simulink model "TCMSSystem"  (R2019b)
settings: configuration reference "ConfigSet_TCMSSystem_Reference" (kept outside this file)
model workspace (MAT data in the model file):
  Prm_TCMSSystem : Simulink.Parameter (value not decoded)
  SampleTime = 0.05
symbols that are objects in the model workspace (value not decoded): Prm_TCMSSystem
undefined symbols (not defined in the file): ADDIntervention, AK1Status, AK2Status, AKContactorStatus, AllDoorsClosed, AllLeftDoorsClosed, AllRightDoorsClosed, APS1Fault, APS1Isolated, APS1OutputVoltage, APS1Status, APS2Fault, APS2Isolated, APS2OutputVoltage, APS2Status, APSKAKContactor, ASCOEnd1, ASCOEnd2, ATBMode, ATCBypassMode, ATCStatusNotOK, ATOMode, ATPLowSpeedCutoutStatus, ATPMode, AuxCompressor, BatteryCurrent, BatteryIsolationContactor, BatteryTemperature, BatteryVoltage, BCG1Fault, BCG1Isolated, BCG1IsolationFailed, BCG1OutputCurrent, BCG1Status, BCG2Fault, BCG2Isolated, BCG2OutputCurrent, BCG2Status, BCGOutputVoltage, BECU1AxleLockedWheelSet1, BECU2AxleLockedWheelSet2, BECUFaulty, BECUMajorFault, BECUMinorFault, BECUStatus, BIC1Inside, BIC1Outside, BIC2Inside, BIC2Outside, Bogie, Bogie1WSPStatus, Bogie2WSPStatus, BogieFaulty, BogieIsolationStatus, BogieSupportedMass, BrakeCylinderPressureGauge, BrakeLoopCBTripped, BrakeLoopOpenTL, BrakeTrainLineStatus, BrakingDemand ... (+215)
libraries: TimersLib x257, simulink x137, LatchesLib x42, VectorOperationsLib x15, TestBenchLib x12, MathOperationsLib x2, FiltersLib x1
(part 4 of 16)

== system TCMSSystem/TCMSSystemPerVehicle/EnabledTCMSVehicle/TCMSPneumatics/PneumaticControl ==
  In Bus Element1 : Inport  PortName=WireStates  Element=TractionBrakingTrainWire.BrakingCommand
  In Bus Element : Inport  Port=2  PortName=IOControl  Element=ASCOEnd1
  In Bus Element2 : Inport  Port=2  PortName=IOControl  Element=ASCOEnd2
  In Bus Element3 : Inport  Port=2  PortName=IOControl  Element=HornManuallyIsolated
  In Bus Element4 : Inport  Port=2  PortName=IOControl  Element=BIC1Inside
  In Bus Element5 : Inport  Port=2  PortName=IOControl  Element=BIC1Outside
  In Bus Element6 : Inport  Port=2  PortName=IOControl  Element=BIC2Inside
  In Bus Element7 : Inport  Port=2  PortName=IOControl  Element=BIC2Outside
  Bus Assignment : BusAssignment  AssignedSignals=BrakingDemand,ASCOEnd1,ASCOEnd2,HornManuallyIsolated,BIC1Inside,BIC1Outside,BIC2Inside,BIC2Outside
  Constant7 : Constant  Value=0  OutDataTypeStr=Bus: BD_TCMSSystem_Out_Vehicle_Control_PneumaticSystem
  Data Type Conversion{,1..6} (7 alike) : DataTypeConversion
  NOT{,1..6} (7 alike) : Logic  Operator=NOT  AllPortsSameDT=off  OutDataTypeStr=boolean
  Control : Outport
  wires:
  Constant7/1 -> Bus Assignment/1  "Control"
  Bus Assignment/1 -> Control/1  "Control"
  In Bus Element1/1 -> Bus Assignment/2
  In Bus Element2/1 -> NOT1/1
  In Bus Element/1 -> NOT/1
  NOT/1 -> Data Type Conversion1/1
  NOT1/1 -> Data Type Conversion/1
  Data Type Conversion/1 -> Bus Assignment/4
  Data Type Conversion1/1 -> Bus Assignment/3
  In Bus Element3/1 -> NOT2/1
  Data Type Conversion2/1 -> Bus Assignment/5
  NOT2/1 -> Data Type Conversion2/1
  NOT3/1 -> Data Type Conversion3/1
  Data Type Conversion3/1 -> Bus Assignment/6
  Data Type Conversion4/1 -> Bus Assignment/7
  NOT4/1 -> Data Type Conversion4/1
  NOT5/1 -> Data Type Conversion5/1
  Data Type Conversion5/1 -> Bus Assignment/8
  Data Type Conversion6/1 -> Bus Assignment/9
  NOT6/1 -> Data Type Conversion6/1
  In Bus Element4/1 -> NOT3/1
  In Bus Element5/1 -> NOT4/1
  In Bus Element6/1 -> NOT5/1
  In Bus Element7/1 -> NOT6/1

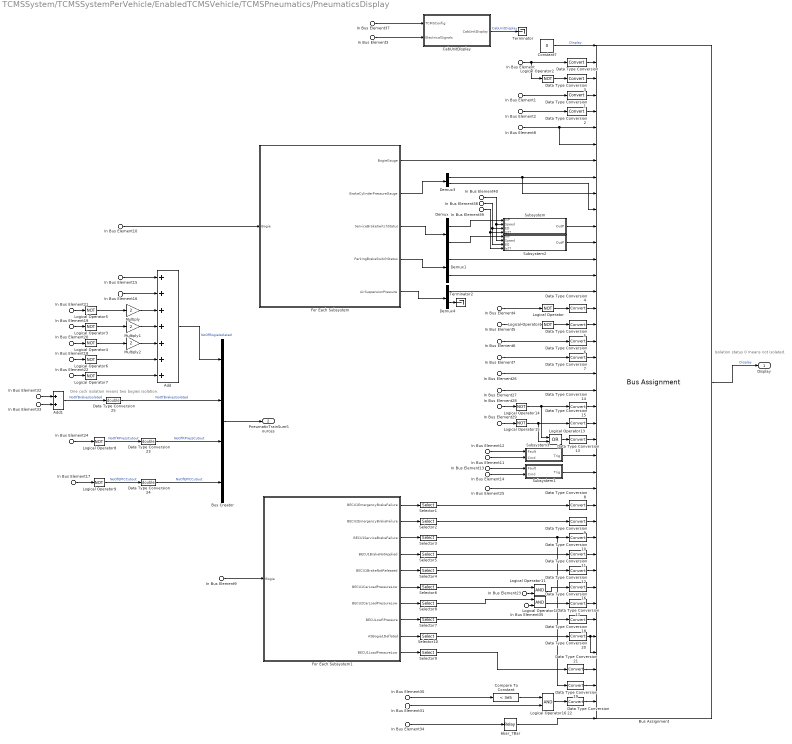
== system TCMSSystem/TCMSSystemPerVehicle/EnabledTCMSVehicle/TCMSPneumatics/PneumaticsDisplay ==
  note: One cock isolation means two bogies isolation.
  note: Isolation status 0 means not isolated.
  In Bus Element37 : Inport  PortName=TCMSSystemVehicleConfig
  In Bus Element39 : Inport  PortName=TCMSSystemVehicleConfig  Element=IsTCar
  In Bus Element3 : Inport  Port=2  PortName=ElectricalSignals
  In Bus Element : Inport  Port=2  PortName=ElectricalSignals  Element=ServiceBrakesReleased
  In Bus Element1 : Inport  Port=2  PortName=ElectricalSignals  Element=ParkBrakesReleased
  In Bus Element2 : Inport  Port=2  PortName=ElectricalSignals  Element=ParkBrakeApplication
  In Bus Element11 : Inport  Port=2  PortName=ElectricalSignals  Element=ParkBrakeApplyCommand
  In Bus Element14 : Inport  Port=2  PortName=ElectricalSignals  Element=ParkBrakeReleaseCommand
  In Bus Element8 : Inport  Port=3  PortName=PneumaticsSystem  Element=MainReservoirPressureGauge
  In Bus Element34 : Inport  Port=3  PortName=PneumaticsSystem  Element=MainReservoirPressureGauge
  In Bus Element10 : Inport  Port=3  PortName=PneumaticsSystem  Element=Bogie
  In Bus Element9 : Inport  Port=3  PortName=PneumaticsSystem  Element=Bogie
  In Bus Element25 : Inport  Port=3  PortName=PneumaticsSystem  Element=BrakeDemandSignalFailure
  In Bus Element30 : Inport  Port=3  PortName=PneumaticsSystem  Element=PantographPressure
  In Bus Element4 : Inport  Port=4  PortName=IOControl  Element=ASCOEnd1
  In Bus Element18 : Inport  Port=4  PortName=IOControl  Element=ASCOEnd1
  In Bus Element5 : Inport  Port=4  PortName=IOControl  Element=ASCOEnd2
  In Bus Element22 : Inport  Port=4  PortName=IOControl  Element=ASCOEnd2
  In Bus Element{6,15,26,32} (4 alike) : Inport  Port=4  PortName=IOControl  Element=Bogie1IsolationCmd
  In Bus Element{7,16,27,33} (4 alike) : Inport  Port=4  PortName=IOControl  Element=Bogie2IsolationCmd
  In Bus Element19 : Inport  Port=4  PortName=IOControl  Element=EPIC
  In Bus Element17 : Inport  Port=4  PortName=IOControl  Element=EPIC
  In Bus Element20 : Inport  Port=4  PortName=IOControl  Element=SR
  In Bus Element24 : Inport  Port=4  PortName=IOControl  Element=SR
  In Bus Element21 : Inport  Port=4  PortName=IOControl  Element=ASIsolationCock
  In Bus Element28 : Inport  Port=4  PortName=IOControl  Element=ParkBrakeIsolationCockBogie1
  In Bus Element29 : Inport  Port=4  PortName=IOControl  Element=ParkBrakeIsolationCockBogie2
  In Bus Element12 : Inport  Port=5  PortName=PneumaticFaults  Element=ParkingBrakeApplicationFailure
  In Bus Element13 : Inport  Port=5  PortName=PneumaticFaults  Element=ParkingBrakeReleaseFailure
  In Bus Element31 : Inport  Port=5  PortName=PneumaticFaults  Element=PantographPipeLowPressure
  In Bus Element23 : Inport  Port=5  PortName=PneumaticFaults  Element=BECU1CarLoadPressureLow
  In Bus Element35 : Inport  Port=5  PortName=PneumaticFaults  Element=BECU2CarLoadPressureLow
  In Bus Element38 : Inport  Port=6  PortName=TractionBrakingFB  Element=EDBrakingCommand
  In Bus Element40 : Inport  Port=7  PortName=Dynamics  Element=VehicleSpeed
  6bar_7Bar : Relay  OnSwitchValue=700000  OffSwitchValue=600000  OnOutputValue=0  OffOutputValue=1
  Add : Sum  Inputs=+++++++
  Add1 : Sum
  Bus Assignment : BusAssignment  AssignedSignals=AllServiceBrakesReleased,ServiceBrakesApplied,AllParkBrakesReleased,ParkBrakeApplied,MainReservoirPressureGauge,MainPipePressure,Bogie,BrakeCylinderPressure,Bogie1BrakeCylinderPressure,Bogie2BrakeCylinderPressure,Bogie1ServiceBrakeStatus,Bogie2ServiceBrakeStatus,Bogie1ParkingBrakeStatus,Bogie2ParkingBrakeStatus,AirSuspensionPressure,Bogie1SUSPStatus,Bogie2SUSPStatus,Bogie1IsolationStatus,Bogie2IsolationStatus,Bogie1ServiceBrakeIsolated,Bogie2ServiceBrakeIsolated,Bogie1ParkingBrakeIsolated,Bogie2ParkingBrakeIsolated,ParkBrakeIsolated,ParkBrakeApplyFailure,ParkBrakeReleaseFailure,BrakeDemandSignalFailure,BECU1EmergencyBrakeFailure,BECU2EmergencyBrakeFailure,BECU1ServiceBrakeFailure,BECU1BrakeNotApplied,BECU1BrakeNotReleased,BECU1CarLoadPressureLow,BECU2CarLoadPressureLow,BECULowRPressure,AirSuspensionBogie1Deflated,Bogie1SUSPFault,BECU1LoadPressureLow,Bogie1ServiceBrakeFault,PantographPipePressureLow,MainReservoirPressureLow
  Bus Creator : BusCreator  Inputs=4  OutDataTypeStr=Bus: BD_TCMSSystem_Wires_PneumaticTrainSum  NonVirtualBus=on
  CabUnitDisplay : Subsystem
  Compare To Constant : simulink/Logic and Bit Operations/Compare To Constant  relop=<  const=3e5  OutDataTypeStr=boolean
  Constant7 : Constant  Value=0  OutDataTypeStr=Bus: BD_TCMSSystem_Out_Vehicle_Display_PneumaticsSystem
  Data Type Conversion{,1..22} (23 alike) : DataTypeConversion
  Data Type Conversion23 : DataTypeConversion  OutDataTypeStr=double
  Data Type Conversion24 : DataTypeConversion  OutDataTypeStr=double
  Data Type Conversion25 : DataTypeConversion  OutDataTypeStr=double
  Demux{,1,3..4} (4 alike) : Demux  Outputs=2
  For Each Subsystem : Subsystem  TreatAsAtomicUnit=on
  For Each Subsystem1 : Subsystem  TreatAsAtomicUnit=on
  Logical Operator{,1..9,14..15} (12 alike) : Logic  Operator=NOT  AllPortsSameDT=off  OutDataTypeStr=boolean
  Logical Operator10 : Logic  AllPortsSameDT=off  OutDataTypeStr=boolean
  Logical Operator11 : Logic  AllPortsSameDT=off  OutDataTypeStr=boolean
  Logical Operator13 : Logic  Operator=OR  AllPortsSameDT=off  OutDataTypeStr=boolean
  Logical Operator16 : Logic  AllPortsSameDT=off  OutDataTypeStr=boolean
  Multiply : Gain  Gain=2
  Multiply1 : Gain  Gain=2
  Multiply2 : Gain  Gain=2
  Selector{1..10} (10 alike) : Selector  InputPortWidth=2  IndexOptions=Index vector (dialog)  Indices=[1]  OutputSizes=1
  Subsystem : Subsystem
  Subsystem1 : Subsystem
  Subsystem2 : Subsystem
  Subsystem3 : Subsystem
  Terminator : Terminator
  Terminator2 : Terminator
  Display : Outport
  PneumaticTrainSumSources : Outport  Port=2
  wires:
  In Bus Element/1 -> Logical Operator2/1, Data Type Conversion/1
  In Bus Element1/1 -> Data Type Conversion1/1
  CabUnitDisplay/1(CabUnitDisplay) -> Terminator/1  "CabUnitDisplay"
  In Bus Element3/1 -> CabUnitDisplay/2(ElectricalSignals)
  In Bus Element37/1 -> CabUnitDisplay/1(TCMSConfig)
  Bus Assignment/1 -> Display/1  "Display"
  Constant7/1 -> Bus Assignment/1  "Display"
  In Bus Element2/1 -> Data Type Conversion2/1
  In Bus Element10/1 -> For Each Subsystem/1(Bogie)
  Logical Operator2/1 -> Data Type Conversion3/1
  Data Type Conversion/1 -> Bus Assignment/2
  Data Type Conversion1/1 -> Bus Assignment/4
  Data Type Conversion2/1 -> Bus Assignment/5
  Data Type Conversion3/1 -> Bus Assignment/3
  For Each Subsystem/3(ServiceBrakeSwitchStatus) -> Demux/1
  For Each Subsystem/4(ParkingBrakeSwitchStatus) -> Demux1/1
  In Bus Element8/1 -> Bus Assignment/7, Bus Assignment/6
  For Each Subsystem/5(AirSuspensionPressure) -> Demux4/1
  Demux4/2 -> Terminator2/1
  Demux/2 -> Subsystem2/1(InP)
  Demux1/1 -> Bus Assignment/14
  Demux1/2 -> Bus Assignment/15
  In Bus Element4/1 -> Logical Operator/1
  In Bus Element5/1 -> Logical Operator1/1
  Demux3/2 -> Bus Assignment/11
  Demux4/1 -> Bus Assignment/16
  Demux3/1 -> Bus Assignment/10, Bus Assignment/9
  Logical Operator/1 -> Data Type Conversion4/1
  Logical Operator1/1 -> Data Type Conversion5/1
  Bus Creator/1 -> PneumaticTrainSumSources/1
  Add/1 -> Bus Creator/1  "NoOfBogieIsolated"
  Data Type Conversion4/1 -> Bus Assignment/17
  Data Type Conversion5/1 -> Bus Assignment/18
  For Each Subsystem/1(BogieGauge) -> Bus Assignment/8
  For Each Subsystem/2(BrakeCylinderPressureGauge) -> Demux3/1
  Subsystem3/1(Trig) -> Bus Assignment/26
  Subsystem1/1(Trig) -> Bus Assignment/27
  In Bus Element13/1 -> Subsystem1/1(Fault)
  In Bus Element12/1 -> Subsystem3/1(Fault)
  In Bus Element14/1 -> Subsystem1/2(Cmd)
  In Bus Element11/1 -> Subsystem3/2(Cmd)
  In Bus Element15/1 -> Add/1
  In Bus Element16/1 -> Add/2
  Logical Operator5/1 -> Multiply/1
  In Bus Element21/1 -> Logical Operator5/1
  Logical Operator3/1 -> Multiply1/1
  Logical Operator4/1 -> Multiply2/1
  In Bus Element20/1 -> Logical Operator4/1
  In Bus Element19/1 -> Logical Operator3/1
  Multiply/1 -> Add/3
  Multiply1/1 -> Add/4
  Multiply2/1 -> Add/5
  Data Type Conversion6/1 -> Bus Assignment/19
  In Bus Element6/1 -> Data Type Conversion6/1
  In Bus Element7/1 -> Data Type Conversion7/1
  Data Type Conversion7/1 -> Bus Assignment/20
  In Bus Element18/1 -> Logical Operator6/1
  In Bus Element22/1 -> Logical Operator7/1
  In Bus Element25/1 -> Bus Assignment/28
  In Bus Element9/1 -> For Each Subsystem1/1(Bogie)
  For Each Subsystem1/1(BECU1EmergencyBrakeFailure) -> Selector1/1
  For Each Subsystem1/2(BECU2EmergencyBrakeFailure) -> Selector2/1
  For Each Subsystem1/3(BECU1ServiceBrakeFailure) -> Selector3/1
  For Each Subsystem1/4(BECU1BrakeNotApplied) -> Selector5/1
  For Each Subsystem1/5(BECU1BrakeNotReleased) -> Selector4/1
  Selector1/1 -> Data Type Conversion8/1
  Selector2/1 -> Data Type Conversion9/1
  Selector3/1 -> Data Type Conversion10/1, Data Type Conversion19/1
  Selector5/1 -> Data Type Conversion11/1
  Selector4/1 -> Data Type Conversion12/1
  Data Type Conversion8/1 -> Bus Assignment/29
  Data Type Conversion9/1 -> Bus Assignment/30
  Data Type Conversion10/1 -> Bus Assignment/31
  Data Type Conversion11/1 -> Bus Assignment/32
  Data Type Conversion12/1 -> Bus Assignment/33
  In Bus Element27/1 -> Bus Assignment/22
  In Bus Element28/1 -> Logical Operator14/1
  In Bus Element29/1 -> Logical Operator15/1
  Logical Operator13/1 -> Data Type Conversion13/1
  Data Type Conversion13/1 -> Bus Assignment/25
  Logical Operator14/1 -> Data Type Conversion14/1, Logical Operator13/1
  Logical Operator15/1 -> Logical Operator13/2, Data Type Conversion15/1
  Data Type Conversion14/1 -> Bus Assignment/23
  Data Type Conversion15/1 -> Bus Assignment/24
  Data Type Conversion17/1 -> Bus Assignment/35
  For Each Subsystem1/8(BECULowRPressure) -> Selector7/1
  For Each Subsystem1/7(BECU2CarLoadPressureLow) -> Selector8/1
  For Each Subsystem1/6(BECU1CarLoadPressureLow) -> Selector6/1
  Selector7/1 -> Data Type Conversion18/1
  Logical Operator10/1 -> Data Type Conversion17/1
  Selector6/1 -> Logical Operator11/1
  Data Type Conversion16/1 -> Bus Assignment/34
  Data Type Conversion18/1 -> Bus Assignment/36
  Data Type Conversion19/1 -> Bus Assignment/40
  Data Type Conversion21/1 -> Bus Assignment/39
  Selector10/1 -> Data Type Conversion20/1
  Selector9/1 -> Data Type Conversion21/1
  For Each Subsystem1/9(ASBogie1Deflated) -> Selector10/1
  For Each Subsystem1/10(BECU1LoadPressureLow) -> Selector9/1
  Data Type Conversion20/1 -> Bus Assignment/38, Bus Assignment/37
  Logical Operator16/1 -> Data Type Conversion22/1
  In Bus Element30/1 -> Compare To Constant/1
  Compare To Constant/1 -> Logical Operator16/1
  In Bus Element31/1 -> Logical Operator16/2
  Data Type Conversion22/1 -> Bus Assignment/41
  Logical Operator6/1 -> Add/6
  Logical Operator7/1 -> Add/7
  In Bus Element34/1 -> 6bar_7Bar/1
  6bar_7Bar/1 -> Bus Assignment/42
  In Bus Element24/1 -> Logical Operator8/1
  Data Type Conversion23/1 -> Bus Creator/3  "NoOfRPressCutout"
  In Bus Element17/1 -> Logical Operator9/1
  Data Type Conversion24/1 -> Bus Creator/4  "NoOfEPICCutout"
  Logical Operator8/1 -> Data Type Conversion23/1  "NoOfRPressCutout"
  Logical Operator9/1 -> Data Type Conversion24/1  "NoOfEPICCutout"
  In Bus Element32/1 -> Add1/1
  In Bus Element33/1 -> Add1/2
  Add1/1 -> Data Type Conversion25/1  "NoOfBrakesIsolated"
  Data Type Conversion25/1 -> Bus Creator/2  "NoOfBrakesIsolated"
  Logical Operator11/1 -> Data Type Conversion16/1
  Selector8/1 -> Logical Operator10/1
  In Bus Element23/1 -> Logical Operator11/2
  In Bus Element35/1 -> Logical Operator10/2
  In Bus Element26/1 -> Bus Assignment/21
  Demux/1 -> Subsystem/1(InP)
  In Bus Element40/1 -> Subsystem2/2(Speed), Subsystem/2(Speed)
  In Bus Element38/1 -> Subsystem2/3(ED), Subsystem/3(ED)
  In Bus Element39/1 -> Subsystem/4(IsT?), Subsystem2/4(IsT?)
  Subsystem/1(OutP) -> Bus Assignment/12
  Subsystem2/1(OutP) -> Bus Assignment/13

== system TCMSSystem/TCMSSystemPerVehicle/EnabledTCMSVehicle/TCMSStatus/TCMSSystemDisplay ==
  TCMSSystemVehicleConfig : Inport
  In Bus Element2 : Inport  Port=2  PortName=DisplayControl  Element=HornIsolate
  In Bus Element1 : Inport  Port=3  PortName=TCMSFaults  Element=CCUCommunicationError
  In Bus Element3 : Inport  Port=3  PortName=TCMSFaults  Element=RIO1Fault
  In Bus Element4 : Inport  Port=3  PortName=TCMSFaults  Element=RIO1RIO2Fault
  In Bus Element5 : Inport  Port=3  PortName=TCMSFaults  Element=ERFault
  In Bus Element7 : Inport  Port=4  PortName=ElectricalIn  Element=MCDR
  AND1 : Logic  AllPortsSameDT=off  OutDataTypeStr=boolean
  Bus Assignment : BusAssignment  AssignedSignals=ConsistSwitchStatusA,ConsistSwitchStatusB,ConsistSwitchStatusC,TrainEthernetRepeaterStatus,TrainBackboneNodeStatus,ECNALGStatus,RemoteHornIsolated,CCUFault,RIO1Fault,RIO1Status,RIO2Status,ERFault,RIO1RIO2Fault
  Bus Selector1 : BusSelector  OutputSignals=HasCab
  Constant : Constant
  Constant1 : Constant
  Constant2 : Constant  Value=0
  Constant7 : Constant  Value=0  OutDataTypeStr=Bus: BD_TCMSSystem_Out_Vehicle_Display_TCMSSystem
  Data Type Conversion : DataTypeConversion
  Data Type Conversion2 : DataTypeConversion
  Switch : Switch  Criteria=u2 > Threshold
  Display : Outport
  wires:
  Constant7/1 -> Bus Assignment/1  "Display"
  Bus Assignment/1 -> Display/1  "Display"
  Constant/1 -> Bus Assignment/7, Bus Assignment/5, Bus Assignment/4, Bus Assignment/3, Bus Assignment/2
  TCMSSystemVehicleConfig/1 -> Bus Selector1/1
  Bus Selector1/1 -> AND1/1  "<HasCab>"
  In Bus Element7/1 -> Data Type Conversion/1
  Data Type Conversion/1 -> Bus Assignment/6
  In Bus Element2/1 -> Bus Assignment/8
  In Bus Element1/1 -> AND1/2
  In Bus Element3/1 -> Bus Assignment/10
  In Bus Element5/1 -> Bus Assignment/13
  AND1/1 -> Data Type Conversion2/1
  Data Type Conversion2/1 -> Bus Assignment/9
  In Bus Element4/1 -> Bus Assignment/14, Switch/2
  Switch/1 -> Bus Assignment/12, Bus Assignment/11
  Constant1/1 -> Switch/3
  Constant2/1 -> Switch/1

== system TCMSSystem/TCMSSystemPerVehicle/EnabledTCMSVehicle/TCMSTractionBraking/HoldingBrakeFB_ASDeflatedExtract ==
  In Bus Element1 : Inport  PortName=WireStates
  In Bus Element : Inport  PortName=WireStates  Element=HoldingBrakeStatus
  In Bus Element3 : Inport  Port=2  PortName=PneumaticsIn  Element=Bogie
  Bus Assignment : BusAssignment  AssignedSignals=HoldingBrakeStatus
  Compare To Constant : simulink/Logic and Bit Operations/Compare To Constant  relop=>=  const=0.8e5  OutDataTypeStr=boolean
  Data Type Conversion : DataTypeConversion
  Demux : Demux  Outputs=2
  For Each Subsystem : Subsystem  TreatAsAtomicUnit=on
  Logical Operator : Logic  AllPortsSameDT=off  OutDataTypeStr=boolean
  Selector : Selector  InputPortWidth=2  IndexOptions=Index vector (dialog)  Indices=1  OutputSizes=1
  Terminator : Terminator
  BusOut : Outport
  ASBogie1Deflated : Outport  Port=2
  wires:
  Bus Assignment/1 -> BusOut/1
  Logical Operator/1 -> Data Type Conversion/1
  In Bus Element1/1 -> Bus Assignment/1
  In Bus Element3/1 -> For Each Subsystem/1(Bogie)
  Demux/2 -> Terminator/1
  Demux/1 -> Compare To Constant/1
  Compare To Constant/1 -> Logical Operator/2
  In Bus Element/1 -> Logical Operator/1
  For Each Subsystem/1(BogieGauge) -> Demux/1
  Data Type Conversion/1 -> Bus Assignment/2
  Selector/1 -> ASBogie1Deflated/1
  For Each Subsystem/2(Out2) -> Selector/1

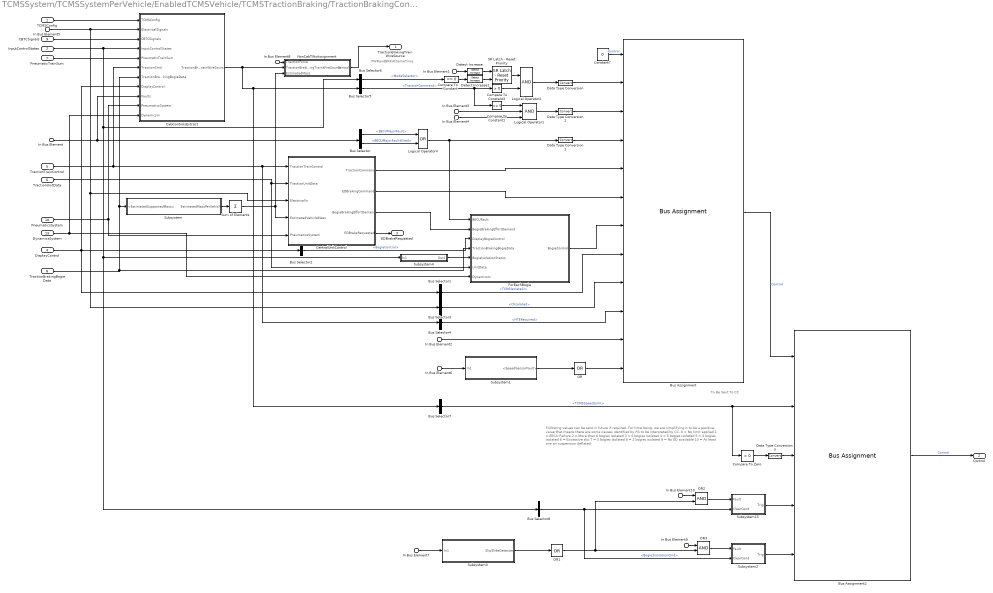
== system TCMSSystem/TCMSSystemPerVehicle/EnabledTCMSVehicle/TCMSTractionBraking/TractionBrakingControl ==
  note: To Be Sent To CC
  note: Following values can be sent in future if required. For time being, we are simplifying it to be a positive value
      | that means there are some causes identified by RS to be interpreted by CC.
      | 0 = No limit applied
      | 1 = EBCU Failure
      | 2 = More than 6 bogies isolated
      | 3 = 6 bogies isolated
      | 4 = 5 bogies isolated
      | 5 = 4 bogies isolated
      | 6 = Excessive slip
      | 7 = 3 bogies isolated
      | 8 = 2 bogies isolated
      | 9 = No ED available
      | 10 = At least one air suspension deflated
  note: PWRandBRKAtSameTime
  TCMSConfig : Inport
  InputControlStates : Inport  Port=2
  In Bus Element5 : Inport  Port=3  PortName=ElectricalSignals
  In Bus Element4 : Inport  Port=3  PortName=ElectricalSignals  Element=CabActive
  DisplayControl : Inport  Port=4
  TractionTrainControl : Inport  Port=5
  TractionUnitData : Inport  Port=6
  PneumaticTrainSum : Inport  Port=7
  TractionBrakingBogieData : Inport  Port=8
  CBTCSignals : Inport  Port=9
  PneumaticsSystem : Inport  Port=10
  In Bus Element : Inport  Port=11  PortName=Faults
  In Bus Element1 : Inport  Port=11  PortName=Faults  Element=BECUPWRAndBRKCmdAtSameTime
  In Bus Element3 : Inport  Port=11  PortName=Faults  Element=TractionCutModeSelectorInATPATOUTO
  In Bus Element2 : Inport  Port=12  PortName=TractionSystem  Element=VehicleDerailed
  In Bus Element6 : Inport  Port=12  PortName=TractionSystem  Element=Bogie
  In Bus Element7 : Inport  Port=12  PortName=TractionSystem  Element=Bogie
  In Bus Element8 : Inport  Port=12  PortName=TractionSystem  Element=TractionForce
  DynamicsSystem : Inport  Port=13
  In Bus Element9 : Inport  Port=14  PortName=VehicleFaults  Element=BECU2AxleLockedWheelSet2
  In Bus Element10 : Inport  Port=14  PortName=VehicleFaults  Element=BECU1AxleLockedWheelSet1
  Bus Assignment : BusAssignment  AssignedSignals=PWRandBRKBothApplied,TractionCutModeSelectorInATPATOUTO,BECUFaulty,TractionCommand,EDBrakingCommand,Bogie,TCMSIsolateCI,CIIsolated,HTERequired,VehicleDerailed,SpeedSensorFault
  Bus Assignment2 : BusAssignment  AssignedSignals=TCMSSpeedLimit,TCMSSpeedLimitCause,BECU1AxleLockedWheelSet1,BECU2AxleLockedWheelSet2
  Bus Selector : BusSelector  OutputSignals=BECUMajorFault,BECUMajorFaultWired
  Bus Selector1 : BusSelector  OutputSignals=TCMSIsolateCI
  Bus Selector2 : BusSelector  OutputSignals=BogieControl
  Bus Selector3 : BusSelector  OutputSignals=CIIsolated
  Bus Selector4 : BusSelector  OutputSignals=HTERequired
  Bus Selector5 : BusSelector  OutputSignals=TractionCommand
  Bus Selector6 : BusSelector  OutputSignals=ModeSelector
  Bus Selector7 : BusSelector  OutputSignals=TCMSSpeedLimit
  Bus Selector8 : BusSelector  OutputSignals=Bogie1IsolationCmd
  CabControlsExtract : Subsystem  TreatAsAtomicUnit=on
  CentralUnitControl : Subsystem  TreatAsAtomicUnit=on
  Compare To Constant : simulink/Logic and Bit Operations/Compare To Constant  relop===  const=0  OutDataTypeStr=boolean
  Compare To Constant1 : simulink/Logic and Bit Operations/Compare To Constant  relop===  const=0  OutDataTypeStr=boolean
  Compare To Constant3 : simulink/Logic and Bit Operations/Compare To Constant  relop=>  const=0  OutDataTypeStr=boolean
  Compare To Zero : simulink/Logic and Bit Operations/Compare To Zero  relop=>  OutDataTypeStr=boolean
  Constant7 : Constant  Value=0  OutDataTypeStr=Bus: BD_TCMSSystem_Out_Vehicle_Control_TractionBraking
  Data Type Conversion{,1..3} (4 alike) : DataTypeConversion
  Detect Increase : simulink/Logic and Bit Operations/Detect Increase  vinit=0.0  OutDataTypeStr=boolean
  Detect Increase1 : simulink/Logic and Bit Operations/Detect Increase  vinit=0.0  OutDataTypeStr=boolean
  ForEachBogie : Subsystem  TreatAsAtomicUnit=on
  Logical Operator1 : Logic  Inputs=3  AllPortsSameDT=off  OutDataTypeStr=boolean
  Logical Operator2 : Logic  AllPortsSameDT=off  OutDataTypeStr=boolean
  Logical Operator4 : Logic  Operator=OR  AllPortsSameDT=off  OutDataTypeStr=boolean
  NonCabTWsAssignment : Subsystem
  OR : Logic  Operator=OR  Inputs=1  AllPortsSameDT=off  OutDataTypeStr=boolean
  OR1 : Logic  Operator=OR  Inputs=1  AllPortsSameDT=off  OutDataTypeStr=boolean
  OR2 : Logic  AllPortsSameDT=off  OutDataTypeStr=boolean
  OR3 : Logic  AllPortsSameDT=off  OutDataTypeStr=boolean
  SR Latch - Reset Priority : LatchesLib/SR Latch - Reset Priority  initial_condition=0
      settings: SourceProductName=Latches
  Subsystem : Subsystem
  Subsystem1 : Subsystem
  Subsystem15 : Subsystem
  Subsystem2 : Subsystem
  Subsystem3 : Subsystem
  Subsystem4 : Subsystem
  Sum of Elements : Sum  Inputs=+
  TractionBrakingTrainWireSource : Outport
  Control : Outport  Port=2
  EDBrakeRequested : Outport  Port=3
  wires:
  Bus Assignment/1 -> Bus Assignment2/1  "Control"
  Constant7/1 -> Bus Assignment/1  "Control"
  TractionTrainControl/1 -> CabControlsExtract/6(TractionCmd), Bus Selector4/1, CentralUnitControl/1(TractionTrainControl)
  Bus Selector2/1 -> ForEachBogie/3(DisplayBogieControl)  "<BogieControl>"
  CentralUnitControl/3(BogieBrakingEffortDemand) -> ForEachBogie/2(BogieBrakingEffortDemand)
  TCMSConfig/1 -> CabControlsExtract/1(TCMSConfig)
  InputControlStates/1 -> Bus Selector8/1, Subsystem4/1(In1), Bus Selector6/1, CabControlsExtract/4(InputControlStates)
  In Bus Element5/1 -> Bus Selector3/1, CentralUnitControl/3(ElectricalIn), CabControlsExtract/2(ElectricalSignals)
  DisplayControl/1 -> Bus Selector1/1, CabControlsExtract/8(DisplayControl), Bus Selector2/1
  CBTCSignals/1 -> CabControlsExtract/3(CBTCSignals)
  CentralUnitControl/4(EDBrakeRequested) -> EDBrakeRequested/1
  CabControlsExtract/1(TractionBrakingTrainWireSource) -> NonCabTWsAssignment/2(TractionBrakingTrainWireSource), Bus Selector5/1, Bus Selector7/1
  TractionBrakingBogieData/1 -> CabControlsExtract/7(TractionBrakingBogieData), Subsystem/1(<EstimatedSupportedMass>), ForEachBogie/4(TractionBrakingBogieData)
  Subsystem/1(EstimatedMassPerVehicle) -> Sum of Elements/1
  Sum of Elements/1 -> CentralUnitControl/4(EstimatedVehicleMass), NonCabTWsAssignment/3(EstimatedMass)
  PneumaticTrainSum/1 -> CabControlsExtract/5(PneumaticTrainSum)
  In Bus Element/1 -> CabControlsExtract/9(Faults), Bus Selector/1
  PneumaticsSystem/1 -> CabControlsExtract/10(PneumaticsSystem), CentralUnitControl/5(PneumaticsSystem)
  Logical Operator4/1 -> Data Type Conversion1/1, ForEachBogie/1(BECUFault)
  Bus Selector/1 -> Logical Operator4/1  "<BECUMajorFault>"
  Bus Selector/2 -> Logical Operator4/2  "<BECUMajorFaultWired>"
  Data Type Conversion/1 -> Bus Assignment/2
  SR Latch - Reset Priority/1 -> Logical Operator2/1
  Detect Increase1/1 -> SR Latch - Reset Priority/2
  Logical Operator2/1 -> Data Type Conversion/1
  In Bus Element1/1 -> Detect Increase/1
  Compare To Constant3/1 -> Logical Operator2/2
  Detect Increase/1 -> SR Latch - Reset Priority/1
  Bus Selector6/1 -> Compare To Constant/1  "<ModeSelector>"
  Compare To Constant/1 -> Detect Increase1/1
  Bus Selector5/1 -> Compare To Constant1/1, Compare To Constant3/1  "<TractionCommand>"
  Compare To Constant1/1 -> Logical Operator1/1
  In Bus Element3/1 -> Logical Operator1/2
  ForEachBogie/1(BogieControl) -> Bus Assignment/7
  CentralUnitControl/2(EDBrakingCommand) -> Bus Assignment/6
  CentralUnitControl/1(TractionCommand) -> Bus Assignment/5
  Data Type Conversion1/1 -> Bus Assignment/4
  Logical Operator1/1 -> Data Type Conversion2/1
  In Bus Element2/1 -> Bus Assignment/11
  Bus Selector4/1 -> Bus Assignment/10  "<HTERequired>"
  Bus Selector3/1 -> Bus Assignment/9  "<CIIsolated>"
  Bus Selector1/1 -> Bus Assignment/8  "<TCMSIsolateCI>"
  Data Type Conversion2/1 -> Bus Assignment/3
  In Bus Element4/1 -> Logical Operator1/3
  Subsystem1/1(<SpeedSensorFault>) -> OR/1
  OR/1 -> Bus Assignment/12
  In Bus Element6/1 -> Subsystem1/1(In1)
  DynamicsSystem/1 -> CabControlsExtract/11(DynamicsIn), ForEachBogie/7(DynamicsIn)
  Bus Assignment2/1 -> Control/1  "Control"
  Compare To Zero/1 -> Data Type Conversion3/1
  Bus Selector7/1 -> Compare To Zero/1, Bus Assignment2/2  "<TCMSSpeedLimit>"
  In Bus Element8/1 -> NonCabTWsAssignment/1(TractionForce)
  NonCabTWsAssignment/1(Control) -> TractionBrakingTrainWireSource/1
  Data Type Conversion3/1 -> Bus Assignment2/3
  Subsystem15/1(Trig) -> Bus Assignment2/4
  Subsystem2/1(Trig) -> Bus Assignment2/5
  In Bus Element9/1 -> OR3/1
  In Bus Element10/1 -> OR2/1
  Bus Selector8/1 -> Subsystem15/2(ClearCond), Subsystem2/2(ClearCond)  "<Bogie1IsolationCmd>"
  In Bus Element7/1 -> Subsystem3/1(In1)
  OR1/1 -> OR2/2, OR3/2
  Subsystem3/1(SlipSlideDetected) -> OR1/1
  OR2/1 -> Subsystem15/1(Fault)
  OR3/1 -> Subsystem2/1(Fault)
  TractionUnitData/1 -> ForEachBogie/6(UnitData), CentralUnitControl/2(TractionUnitData)
  Subsystem4/1(Out1) -> ForEachBogie/5(BogieIsolationStatus)

== system TCMSSystem/TCMSSystemPerVehicle/EnabledTCMSVehicle/TCMSTractionBraking/TractionBrakingDataExtract ==
  note: Summing bogie outputs on each vehicle
  note: TCMSTractionVehicle
  TCMSSystemVehicleConfig : Inport
  In Bus Element : Inport  Port=2  PortName=TractionSystem  Element=Bogie
  In Bus Element2 : Inport  Port=2  PortName=TractionSystem  Element=TCU_KStatus
  In Bus Element3 : Inport  Port=2  PortName=TractionSystem  Element=TCU_AKStatus
  In Bus Element1 : Inport  Port=3  PortName=PneumaticsSystem  Element=Bogie
  AND : Logic  AllPortsSameDT=off  OutDataTypeStr=boolean
  AND1 : Logic  AllPortsSameDT=off  OutDataTypeStr=boolean
  Abs : Abs
  Abs1 : Abs
  Bus Creator : BusCreator  Inputs=13  OutDataTypeStr=Bus: BD_TCMSSystem_Wires_TBUnitSum  NonVirtualBus=on
  Bus Creator1 : BusCreator  Inputs=5  OutDataTypeStr=Bus: BD_TCMSSystem_Wires_TBUnitWire  NonVirtualBus=on
  Bus Selector : BusSelector  OutputSignals=NumberOfTractionBogies,NumberOfBrakingBogies
  Compare To Zero : simulink/Logic and Bit Operations/Compare To Zero  relop=>  OutDataTypeStr=boolean
  Compare To Zero1 : simulink/Logic and Bit Operations/Compare To Zero  relop=>  OutDataTypeStr=boolean
  Compare To Zero2 : simulink/Logic and Bit Operations/Compare To Zero  relop=>  OutDataTypeStr=boolean
  Data Type Conversion{,1..4} (5 alike) : DataTypeConversion
  Gain : Gain
  Gain1 : Gain
  NOT : Logic  Operator=NOT  AllPortsSameDT=off  OutDataTypeStr=boolean
  OR : Logic  Operator=OR  AllPortsSameDT=off  OutDataTypeStr=boolean
  OR1 : Logic  Operator=OR  Inputs=1  AllPortsSameDT=off  OutDataTypeStr=boolean
  OR3 : Logic  Operator=OR  Inputs=1  AllPortsSameDT=off  OutDataTypeStr=boolean
  OR4 : Logic  Operator=OR  Inputs=1  AllPortsSameDT=off  OutDataTypeStr=boolean
  Subsystem : Subsystem
  Sum of Elements{,1..10} (11 alike) : Sum  Inputs=+
  TCMSTractionBogie : Subsystem
  TractionBrakingVehicleData : Outport
  TractionBrakingBogieData : Outport  Port=2
  TractionBrakingUnitWireSources : Outport  Port=3
  wires:
  In Bus Element/1 -> TCMSTractionBogie/1(TractionBogieSignals)  "BogieSignals"
  TCMSTractionBogie/1(TCMSBogieData) -> [BogieData], TractionBrakingBogieData/1
  TCMSTractionBogie/11(TractionBogieAvailable) -> Sum of Elements8/1, OR1/1
  TCMSTractionBogie/2(BogieTractiveEffortAchieved) -> Sum of Elements7/1
  TCMSTractionBogie/3(BogieEDBrakingEffortAchieved) -> Sum of Elements6/1
  TCMSTractionBogie/4(BogieTractiveEffortPossible) -> Sum of Elements5/1
  TCMSTractionBogie/5(BogieEDBrakingEffortPossible) -> Sum of Elements4/1
  TCMSTractionBogie/6(BogieTractivePowerAchieved) -> Sum of Elements3/1
  TCMSTractionBogie/7(BogieEDBrakingPowerAchieved) -> Sum of Elements2/1
  TCMSTractionBogie/8(BogieTractivePowerPossible) -> Sum of Elements1/1
  TCMSTractionBogie/9(BogieEDBrakingPowerPossible) -> Sum of Elements/1
  Sum of Elements/1 -> Bus Creator/10  "EDBrakingPowerPossible"
  Sum of Elements1/1 -> Bus Creator/9  "TractivePowerPossible"
  Sum of Elements2/1 -> Bus Creator/8  "EDBrakingPowerAchieved"
  Sum of Elements3/1 -> Bus Creator/7  "TractivePowerAchieved"
  Sum of Elements4/1 -> Bus Creator/6  "EDBrakingEffortPossible"
  Sum of Elements5/1 -> Bus Creator/5  "TractiveEffortPossible"
  Sum of Elements6/1 -> Bus Creator/4, [EDBrakingEffortAchieved]  "EDBrakingEffortAchieved"
  Sum of Elements7/1 -> Bus Creator/3, [TractiveEffortAchieved]  "TractiveEffortAchieved"
  Sum of Elements8/1 -> Bus Creator/12  "TractionBogiesAvailable"
  Bus Creator/1 -> TractionBrakingVehicleData/1
  In Bus Element1/1 -> TCMSTractionBogie/2(PneumaticsBogieSignals)  "BogieSignals"
  TCMSTractionBogie/10(EstimatedBogieSupportedMass) -> Sum of Elements9/1
  Sum of Elements9/1 -> Bus Creator/11  "EstimatedMass"
  TCMSTractionBogie/12(EDBrakingBogieAvailable) -> Sum of Elements10/1
  Sum of Elements10/1 -> Bus Creator/13  "EDBrakingBogiesAvailable"
  TCMSSystemVehicleConfig/1 -> Bus Selector/1
  Bus Selector/1 -> Gain/1  "<NumberOfTractionBogies>"
  Bus Selector/2 -> Gain1/1  "<NumberOfBrakingBogies>"
  Gain/1 -> Bus Creator/1  "TractionBogiesEquipped"
  Gain1/1 -> Bus Creator/2  "BrakingBogiesEquipped"
  [TractiveEffortAchieved] -> Abs/1
  [EDBrakingEffortAchieved] -> Abs1/1
  Compare To Zero/1 -> OR/1
  Compare To Zero1/1 -> OR/2
  Data Type Conversion2/1 -> Bus Creator1/3  "PropulsionActive"
  OR1/1 -> NOT/1
  TCMSTractionBogie/13(BogieFaulty) -> OR4/1
  OR4/1 -> Compare To Zero2/1
  Data Type Conversion1/1 -> Bus Creator1/2  "PropulsionFault"
  Data Type Conversion/1 -> Bus Creator1/1  "PropulsionIsolated"
  Compare To Zero2/1 -> Data Type Conversion1/1
  OR/1 -> Data Type Conversion2/1
  Data Type Conversion3/1 -> Bus Creator1/4  "PropulsionEnabled"
  [BogieData] -> Subsystem/1(BogieData)
  Subsystem/1(<TCUStatus>) -> OR3/1
  OR3/1 -> AND/2, Data Type Conversion3/1
  AND/1 -> Data Type Conversion/1
  In Bus Element2/1 -> AND1/1
  In Bus Element3/1 -> AND1/2
  AND1/1 -> Data Type Conversion4/1
  Data Type Conversion4/1 -> Bus Creator1/5  "CI_K_AK_Status"
  Bus Creator1/1 -> TractionBrakingUnitWireSources/1
  NOT/1 -> AND/1
  Abs/1 -> Compare To Zero/1
  Abs1/1 -> Compare To Zero1/1

== system TCMSSystem/TCMSSystemPerVehicle/EnabledTCMSVehicle/TCMSTractionBraking/TractionBrakingDisplay ==
  In Bus Element2 : Inport  PortName=TCMSSystemVehicleConfig
  In Bus Element22 : Inport  Port=2  PortName=IOControl
  In Bus Element8 : Inport  Port=2  PortName=IOControl
  In Bus Element{,1,13,16,28} (5 alike) : Inport  Port=3  PortName=ElectricalSignals
  In Bus Element6 : Inport  Port=4  PortName=TractionBrakingTW
  In Bus Element12 : Inport  Port=4  PortName=TractionBrakingTW
  In Bus Element19 : Inport  Port=4  PortName=TractionBrakingTW
  In Bus Element21 : Inport  Port=5  PortName=TractionUnitData
  In Bus Element15 : Inport  Port=6  PortName=PneumaticTrainSum
  In Bus Element20 : Inport  Port=7  PortName=CBTC
  In Bus Element5 : Inport  Port=8  PortName=TractionVehicleData
  In Bus Element7 : Inport  Port=8  PortName=TractionVehicleData
  In Bus Element10 : Inport  Port=9  PortName=TractionOnBogieData
  In Bus Element9 : Inport  Port=9  PortName=TractionOnBogieData
  In Bus Element3 : Inport  Port=10  PortName=TractionBrakingUnitData
  In Bus Element14 : Inport  Port=11  PortName=TractionBrakingUW
  In Bus Element4 : Inport  Port=12  PortName=TractionSystem
  In Bus Element11 : Inport  Port=13  PortName=BrakingSystem
  In Bus Element17 : Inport  Port=14  PortName=Faults
  In Bus Element18 : Inport  Port=15  PortName=VehicleFaults
  In Bus Element23 : Inport  Port=15  PortName=VehicleFaults
  In Bus Element24 : Inport  Port=16  PortName=DisplayControl
  BrakeScreen : Subsystem
  Constant7 : Constant  Value=0  OutDataTypeStr=Bus: BD_TCMSSystem_Out_Vehicle_Display_TractionBraking
  HVScreen : Subsystem
  OperatingandOtherScreen : Subsystem
  PropulsionScreen : Subsystem
  SpeedLimitationInterlockScreen : Subsystem
  Display : Outport
  wires:
  [SlipDetected] -> SpeedLimitationInterlockScreen/6(SlipDetected)
  SpeedLimitationInterlockScreen/1(Display) -> HVScreen/1(BusIn)  "Display"
  In Bus Element28/1 -> SpeedLimitationInterlockScreen/3(ElectricalSignals)
  In Bus Element22/1 -> SpeedLimitationInterlockScreen/2(IOControls)
  PropulsionScreen/1(BusOut) -> SpeedLimitationInterlockScreen/1(BusIn)
  In Bus Element3/1 -> PropulsionScreen/2(TractionBrakingUnitData)
  In Bus Element4/1 -> PropulsionScreen/3(TractionSystem)
  BrakeScreen/1(BusOut) -> PropulsionScreen/1(BusIn)
  In Bus Element7/1 -> BrakeScreen/4(TractionVehicleData)
  In Bus Element6/1 -> BrakeScreen/2(TractionBrakingTW)
  In Bus Element8/1 -> BrakeScreen/3(IOControl)
  In Bus Element10/1 -> BrakeScreen/5(TractionOnBogieData)
  In Bus Element11/1 -> BrakeScreen/6(BrakingSystem)
  In Bus Element1/1 -> BrakeScreen/7(ElectricalSignals)
  OperatingandOtherScreen/1(BusOut) -> BrakeScreen/1(BusIn)
  In Bus Element2/1 -> OperatingandOtherScreen/2(TCMSSystemVehicleConfig)
  In Bus Element/1 -> OperatingandOtherScreen/3(ElectricalSignals)
  In Bus Element21/1 -> OperatingandOtherScreen/4(TractionUnitData)
  In Bus Element5/1 -> OperatingandOtherScreen/5(TractionVehicleData)
  In Bus Element14/1 -> HVScreen/3(TractionBrakingUW)
  In Bus Element12/1 -> OperatingandOtherScreen/6(TractionBrakingTW)
  Constant7/1 -> OperatingandOtherScreen/1(BusIn)  "Display"
  In Bus Element15/1 -> SpeedLimitationInterlockScreen/4(PneumaticTrainSum)
  In Bus Element9/1 -> PropulsionScreen/4(TractionOnBogieData)
  In Bus Element17/1 -> BrakeScreen/8(Faults)
  In Bus Element16/1 -> PropulsionScreen/5(ElectricalFB)
  In Bus Element18/1 -> PropulsionScreen/6(VehicleFault)
  In Bus Element20/1 -> PropulsionScreen/7(CBTC)
  In Bus Element19/1 -> PropulsionScreen/8(TractionTW)
  HVScreen/1(Display) -> Display/1  "Display"
  In Bus Element13/1 -> HVScreen/2(ElectricalSignals)
  In Bus Element23/1 -> BrakeScreen/9(VehicleFaults)
  In Bus Element24/1 -> SpeedLimitationInterlockScreen/5(DisplayControl)

== system TCMSSystem/TCMSSystemPerVehicle/LimpHomeTCMSVehicle/CabUnitDisplay/CabActiveUnitDisplay ==
  In Bus Element : Inport  PortName=ElectricalSignals  Element=HMIPower
  Action Port : ActionPort  ActionPortLabel=if(u1 > 0)
  Bus Creator : BusCreator  Inputs=1
  Data Type Conversion : DataTypeConversion  OutDataTypeStr=double
  Out1 : Outport
  wires:
  Data Type Conversion/1 -> Bus Creator/1  "HMIPower"
  In Bus Element/1 -> Data Type Conversion/1
  Bus Creator/1 -> Out1/1

== system TCMSSystem/TCMSSystemPerVehicle/LimpHomeTCMSVehicle/TCMSTractionBraking/TractionBrakingControl ==
  TCMSConfig : Inport
  InputControlStates : Inport  Port=2
  ElectricalSignals : Inport  Port=3
  DisplayControl : Inport  Port=4
  TractionTrainControl : Inport  Port=5
  TractionUnitData : Inport  Port=6
  PneumaticTrainSum : Inport  Port=7
  TractionBrakingBogieData : Inport  Port=8
  CBTCSignals : Inport  Port=9
  Bus Assignment : BusAssignment  AssignedSignals=TractionCommand,EDBrakingCommand,Bogie
  CabControlsExtract : Subsystem  TreatAsAtomicUnit=on
  CentralUnitControl : Subsystem  TreatAsAtomicUnit=on
  Constant7 : Constant  Value=0  OutDataTypeStr=Bus: BD_TCMSSystem_Out_Vehicle_Control_TractionBraking
  ForEachBogie : Subsystem  TreatAsAtomicUnit=on
  TractionBrakingTrainWireSource : Outport
  Control : Outport  Port=2
  wires:
  Bus Assignment/1 -> Control/1  "Control"
  Constant7/1 -> Bus Assignment/1  "Control"
  CentralUnitControl/1(TractionCommand) -> Bus Assignment/2
  CentralUnitControl/2(EDBrakingCommand) -> Bus Assignment/3
  TractionTrainControl/1 -> CabControlsExtract/7(TractionCmd), CentralUnitControl/1(TractionTrainControl)
  TractionUnitData/1 -> CentralUnitControl/2(TractionUnitData)
  ForEachBogie/1(BogieControl) -> Bus Assignment/4
  CentralUnitControl/3(BogieBrakingEffortDemand) -> ForEachBogie/1(BogieBrakingEffortDemand)
  TCMSConfig/1 -> CabControlsExtract/1(TCMSConfig)
  InputControlStates/1 -> CabControlsExtract/5(InputControlStates)
  ElectricalSignals/1 -> CabControlsExtract/2(ElectricalSignals)
  DisplayControl/1 -> CabControlsExtract/3(DisplayControl)
  CabControlsExtract/1(TractionBrakingTrainWireSource) -> TractionBrakingTrainWireSource/1
  CBTCSignals/1 -> CabControlsExtract/4(CBTCSignals)
  TractionBrakingBogieData/1 -> ForEachBogie/2(TractionBrakingBogieData)
  PneumaticTrainSum/1 -> CabControlsExtract/6(PneumaticTrainSum)

== system TCMSSystem/TCMSSystemPerVehicle/LimpHomeTCMSVehicle/TCMSTractionBraking/TractionBrakingDataExtract ==
  note: Summing bogie outputs on each vehicle
  note: TCMSTractionVehicle
  TCMSSystemVehicleConfig : Inport
  In Bus Element : Inport  Port=2  PortName=TractionSystem  Element=Bogie
  In Bus Element2 : Inport  Port=2  PortName=TractionSystem  Element=TCU_KStatus
  In Bus Element3 : Inport  Port=2  PortName=TractionSystem  Element=TCU_AKStatus
  AND : Logic  AllPortsSameDT=off  OutDataTypeStr=boolean
  AND1 : Logic  Operator=OR  AllPortsSameDT=off  OutDataTypeStr=boolean
  Bus Creator : BusCreator  Inputs=13  OutDataTypeStr=Bus: BD_TCMSSystem_Wires_TBUnitSum  NonVirtualBus=on
  Bus Creator1 : BusCreator  Inputs=5  OutDataTypeStr=Bus: BD_TCMSSystem_Wires_TBUnitWire  NonVirtualBus=on
  Bus Selector : BusSelector  OutputSignals=NumberOfTractionBogies,NumberOfBrakingBogies
  Compare To Zero : simulink/Logic and Bit Operations/Compare To Zero  relop=>  OutDataTypeStr=boolean
  Compare To Zero1 : simulink/Logic and Bit Operations/Compare To Zero  relop=>  OutDataTypeStr=boolean
  Compare To Zero2 : simulink/Logic and Bit Operations/Compare To Zero  relop=>  OutDataTypeStr=boolean
  Data Type Conversion{,1..4} (5 alike) : DataTypeConversion
  Gain : Gain
  Gain1 : Gain
  NAND : Logic  Operator=NAND  AllPortsSameDT=off  OutDataTypeStr=boolean
  OR : Logic  Operator=OR  AllPortsSameDT=off  OutDataTypeStr=boolean
  OR{1..2,4..5} (4 alike) : Logic  Operator=OR  Inputs=1  AllPortsSameDT=off  OutDataTypeStr=boolean
  Subsystem : Subsystem
  Sum of Elements{,1..10} (11 alike) : Sum  Inputs=+
  TCMSTractionBogie : Subsystem
  TractionBrakingVehicleData : Outport
  TractionBrakingBogieData : Outport  Port=2
  TractionBrakingUnitWireSources : Outport  Port=3
  wires:
  In Bus Element/1 -> TCMSTractionBogie/1(TractionBogieSignals)  "BogieSignals"
  TCMSTractionBogie/1(TCMSBogieData) -> [BogieData], TractionBrakingBogieData/1
  TCMSTractionBogie/11(TractionBogieAvailable) -> Sum of Elements8/1, OR1/1
  TCMSTractionBogie/2(BogieTractiveEffortAchieved) -> Sum of Elements7/1
  TCMSTractionBogie/3(BogieEDBrakingEffortAchieved) -> Sum of Elements6/1
  TCMSTractionBogie/4(BogieTractiveEffortPossible) -> Sum of Elements5/1
  TCMSTractionBogie/5(BogieEDBrakingEffortPossible) -> Sum of Elements4/1
  TCMSTractionBogie/6(BogieTractivePowerAchieved) -> Sum of Elements3/1
  TCMSTractionBogie/7(BogieEDBrakingPowerAchieved) -> Sum of Elements2/1
  TCMSTractionBogie/8(BogieTractivePowerPossible) -> Sum of Elements1/1
  TCMSTractionBogie/9(BogieEDBrakingPowerPossible) -> Sum of Elements/1
  Sum of Elements/1 -> Bus Creator/10  "EDBrakingPowerPossible"
  Sum of Elements1/1 -> Bus Creator/9  "TractivePowerPossible"
  Sum of Elements2/1 -> Bus Creator/8  "EDBrakingPowerAchieved"
  Sum of Elements3/1 -> Bus Creator/7  "TractivePowerAchieved"
  Sum of Elements4/1 -> Bus Creator/6  "EDBrakingEffortPossible"
  Sum of Elements5/1 -> Bus Creator/5  "TractiveEffortPossible"
  Sum of Elements6/1 -> Bus Creator/4, [EDBrakingEffortAchieved]  "EDBrakingEffortAchieved"
  Sum of Elements7/1 -> Bus Creator/3, [TractiveEffortAchieved]  "TractiveEffortAchieved"
  Sum of Elements8/1 -> Bus Creator/12  "TractionBogiesAvailable"
  Bus Creator/1 -> TractionBrakingVehicleData/1
  TCMSTractionBogie/10(EstimatedBogieSupportedMass) -> Sum of Elements9/1
  Sum of Elements9/1 -> Bus Creator/11  "EstimatedMass"
  TCMSTractionBogie/12(EDBrakingBogieAvailable) -> OR2/1, Sum of Elements10/1
  Sum of Elements10/1 -> Bus Creator/13  "EDBrakingBogiesAvailable"
  TCMSSystemVehicleConfig/1 -> Bus Selector/1
  Bus Selector/1 -> Gain/1  "<NumberOfTractionBogies>"
  Bus Selector/2 -> Gain1/1  "<NumberOfBrakingBogies>"
  Gain/1 -> Bus Creator/1  "TractionBogiesEquipped"
  Gain1/1 -> Bus Creator/2  "BrakingBogiesEquipped"
  [TractiveEffortAchieved] -> Compare To Zero/1
  [EDBrakingEffortAchieved] -> Compare To Zero1/1
  Compare To Zero/1 -> OR/1
  Compare To Zero1/1 -> OR/2
  Data Type Conversion2/1 -> Bus Creator1/3  "PropulsionActive"
  NAND/1 -> AND/1
  TCMSTractionBogie/13(BogieFaulty) -> OR4/1
  OR4/1 -> Compare To Zero2/1
  Data Type Conversion1/1 -> Bus Creator1/2  "PropulsionFault"
  OR1/1 -> NAND/1
  OR2/1 -> NAND/2
  Data Type Conversion/1 -> Bus Creator1/1  "PropulsionIsolated"
  Compare To Zero2/1 -> Data Type Conversion1/1  "PropulsionFault"
  OR/1 -> Data Type Conversion2/1
  Data Type Conversion3/1 -> Bus Creator1/4  "PropulsionEnabled"
  [BogieData] -> Subsystem/1(BogieData)
  Subsystem/1(<TCUStatus>) -> OR5/1
  OR5/1 -> AND/2, Data Type Conversion3/1
  AND/1 -> Data Type Conversion/1
  AND1/1 -> Data Type Conversion4/1
  In Bus Element3/1 -> AND1/2
  In Bus Element2/1 -> AND1/1
  Data Type Conversion4/1 -> Bus Creator1/5  "CI_K_AK_Status"
  Bus Creator1/1 -> TractionBrakingUnitWireSources/1

== system TCMSSystem/TCMSSystemPerVehicle/EnabledTCMSVehicle/OutputsPacking/TCMSDisplayOutputs/TCMSMessageEvents ==
  In Bus Element{,1..2,9,11..12,15..16,26} (9 alike) : Inport  PortName=BusIn
  In Bus Element8 : Inport  Port=2  PortName=TCMSFaults
  In Bus Element14 : Inport  Port=2  PortName=TCMSFaults
  In Bus Element28 : Inport  Port=3  PortName=PneumaticsControl
  In Bus Element{4,6..7,10,13} (5 alike) : Inport  Port=4  PortName=VehicleLevelFaults
  In Bus Element{17..18,21..24,27} (7 alike) : Inport  Port=5  PortName=ElectricalControl
  In Bus Element19 : Inport  Port=6  PortName=DoorsControl
  In Bus Element{3,5,20,25} (4 alike) : Inport  Port=7  PortName=TractionControl
  BrakeSystemFaults : Subsystem
  Bus Assignment : BusAssignment  AssignedSignals=MessageList
  Bus Creator : BusCreator  Inputs=1  OutDataTypeStr=Bus: BD_TCMSSystem_Out_Vehicle_Display_MessageList  NonVirtualBus=on
  DoorSystemFaults : Subsystem
  ElectricalSystemFaults : Subsystem
  MessageShortList : Subsystem
  MiscellaneousFaults : Subsystem
  New46EventsMessage : Subsystem
  PantographSystemFaults : Subsystem
  TCMSSystemFaults : Subsystem
  TractionSystemFaults : Subsystem
  BusOut : Outport
  wires:
  MessageShortList/1(ActiveFaults) -> Bus Creator/1  "Message"
  Bus Creator/1 -> Bus Assignment/2
  Bus Assignment/1 -> BusOut/1
  In Bus Element/1 -> Bus Assignment/1
  In Bus Element9/1 -> DoorSystemFaults/1(BusIn)
  DoorSystemFaults/1(MessageOut) -> TractionSystemFaults/1(MessageIn)
  TractionSystemFaults/1(MessageOut) -> ElectricalSystemFaults/1(MessageIn)
  ElectricalSystemFaults/1(MessageOut) -> BrakeSystemFaults/1(MessageIn)
  BrakeSystemFaults/1(MessageOut) -> TCMSSystemFaults/1(MessageIn)
  TCMSSystemFaults/1(MessageOut) -> MiscellaneousFaults/1(MessageIn)
  MiscellaneousFaults/1(MessageOut) -> PantographSystemFaults/1(MessageIn)
  New46EventsMessage/1(MessageOut) -> MessageShortList/1(AllFaults)
  In Bus Element8/1 -> TCMSSystemFaults/3(TCMSFaults)
  In Bus Element1/1 -> ElectricalSystemFaults/2(BusIn)
  In Bus Element2/1 -> PantographSystemFaults/2(BusIn)
  In Bus Element6/1 -> TractionSystemFaults/3(VehicleLevelFaults)
  In Bus Element7/1 -> ElectricalSystemFaults/3(VehicleLevelFaults)
  In Bus Element10/1 -> BrakeSystemFaults/5(VehicleLevelFaults)
  In Bus Element13/1 -> MiscellaneousFaults/2(VehicleLevelFaults)
  In Bus Element12/1 -> BrakeSystemFaults/2(BusIn)
  In Bus Element15/1 -> TCMSSystemFaults/2(BusIn)
  In Bus Element16/1 -> MiscellaneousFaults/3(BusIn)
  In Bus Element17/1 -> ElectricalSystemFaults/4(ElectricalControl)
  In Bus Element18/1 -> TractionSystemFaults/4(ElectricalControl)
  In Bus Element11/1 -> TractionSystemFaults/2(BusIn)
  In Bus Element19/1 -> DoorSystemFaults/2(DoorsControl)
  In Bus Element3/1 -> TractionSystemFaults/5(TractionControl)
  In Bus Element4/1 -> DoorSystemFaults/3(VehicleFaults)
  In Bus Element5/1 -> BrakeSystemFaults/3(TractionControl)
  In Bus Element14/1 -> BrakeSystemFaults/4(TCMSFaults)
  In Bus Element20/1 -> MiscellaneousFaults/4(TractionControl)
  In Bus Element21/1 -> MiscellaneousFaults/5(ElectricalControl)
  In Bus Element22/1 -> TCMSSystemFaults/4(ElectricalControl)
  In Bus Element23/1 -> DoorSystemFaults/4(ElectricalControl)
  In Bus Element24/1 -> BrakeSystemFaults/6(ElectricalControl)
  In Bus Element25/1 -> TCMSSystemFaults/5(TractionControl)
  PantographSystemFaults/1(MessageOut) -> New46EventsMessage/1(MessageIn)
  In Bus Element26/1 -> New46EventsMessage/2(BusIn)
  In Bus Element27/1 -> New46EventsMessage/3(ElectricalControl)
  In Bus Element28/1 -> New46EventsMessage/4(PneumaticsControl)

== system TCMSSystem/TCMSSystemPerVehicle/EnabledTCMSVehicle/TCMSDoors/CabControlsExtract/CabActiveTrainControl ==
  CBTC : Inport
  Action Port : ActionPort  ActionPortLabel=if(u1 > 0)
  Bus Creator : BusCreator  Inputs=4  OutDataTypeStr=Bus: BD_TCMSSystem_Wires_DoorsTrainWire  NonVirtualBus=on
  Bus Selector : BusSelector  OutputSignals=LeftDoorOpenRequest,RightDoorOpenRequest,LeftDoorCloseRequest,RightDoorCloseRequest
  Out1 : Outport
  wires:
  Bus Creator/1 -> Out1/1
  CBTC/1 -> Bus Selector/1  "CBTC"
  Bus Selector/1 -> Bus Creator/1  "<LeftDoorOpenRequest>"
  Bus Selector/2 -> Bus Creator/2  "<RightDoorOpenRequest>"
  Bus Selector/3 -> Bus Creator/3  "<LeftDoorCloseRequest>"
  Bus Selector/4 -> Bus Creator/4  "<RightDoorCloseRequest>"

== system TCMSSystem/TCMSSystemPerVehicle/EnabledTCMSVehicle/TCMSDoors/CabControlsExtract/CabInactiveNoTrainControl ==
  Action Port : ActionPort  ActionPortLabel=else
  Constant3 : Constant  Value=0  OutDataTypeStr=Bus: BD_TCMSSystem_Wires_DoorsTrainWire
  Out1 : Outport
  wires:
  Constant3/1 -> Out1/1

== system TCMSSystem/TCMSSystemPerVehicle/EnabledTCMSVehicle/TCMSDoors/DoorsControl/For Each Subsystem4 ==
  Source1 : Inport  Partition=on  PartitionDimension=1  PartitionWidth=1  PartitionOffset=0
  Source2 : Inport  Port=2  Partition=on  PartitionDimension=1  PartitionWidth=1  PartitionOffset=0
  Orientation : Inport  Port=3
  For Each : ForEach  DisableCoverage=on
  Orientation Swap : VectorOperationsLib/Orientation Swap
      settings: SourceProductName=Sydac Utilities
  WireState1 : Outport  ConcatenationDimension=1
  WireState2 : Outport  Port=2  ConcatenationDimension=1
  wires:
  Source1/1 -> Orientation Swap/1
  Orientation Swap/1 -> WireState1/1
  Orientation Swap/2 -> WireState2/1
  Source2/1 -> Orientation Swap/2
  Orientation/1 -> Orientation Swap/3
